simulink model "stateflow_function"  (R2015b)
settings: Solver=VariableStepAuto  StartTime=0.0  StopTime=10.0  RelTol=1e-3
settings Model: Creator=amyyang  LastModifiedBy=amyyang

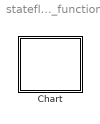
== system stateflow_function ==
  Chart : Stateflow chart  TreatAsAtomicUnit=on

== stateflow chart stateflow_function/Chart ==
  note: 不要直接把函数作为比较对象
  note: 这样相互比较的数据类型明显
  state temp_k = temp_test [function]
  (junction 1) -> (junction 2) : {
      |   a = tem_test();
      | }
  (junction 75) -> (junction 67)
  (junction 2) -> (junction 36) [order 1] : [ a == 1]
  (junction 67) -> (junction 72) [order 1] : [ tem_test() == 1]
  (junction 2) -> (junction 40) [order 2] : {
      | d = b + c;
      | }
  (junction 36) -> (junction 38)
  (junction 67) -> (junction 66) [order 2] : {
      | d = b + c;
      | }
  (junction 72) -> (junction 70)
  (junction 38) -> (junction 40)
  (junction 70) -> (junction 66)
  (junction 40) -> (junction 62)
  (junction 66) -> (junction 73)
  data: temp_k function_output double
